simulink model "basic_electricalcircuit"  (R2019a)
settings: Solver=VariableStepAuto  StartTime=0.0  StopTime=0.01  RelTol=1e-3
libraries: powerlib x5
settings Model: Creator=Deepak  LastModifiedBy=Deepak

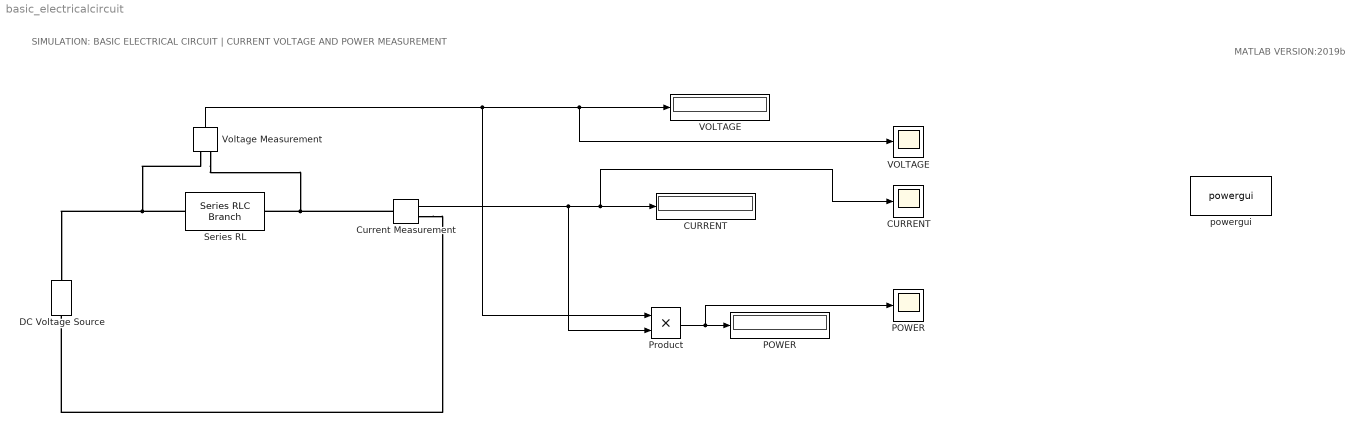
== system basic_electricalcircuit ==
  note: MATLAB VERSION:2019b
  note: SIMULATION: BASIC ELECTRICAL CIRCUIT | CURRENT VOLTAGE AND POWER MEASUREMENT
  CURRENT : Scope
  "CURRENT " : Display
  Current Measurement : powerlib/Measurements/Current Measurement  PhasorSimulation=off  OutputType=Complex  PSBequivalent=0
      settings: SourceProductName=Simscape Electrical
  "DC Voltage Source " : powerlib/Electrical Sources/DC Voltage Source  Amplitude=100  Measurements=None
      settings: SourceProductName=Simscape Electrical
  POWER : Scope
  "POWER " : Display
  Product : Product
  "Series RL " : powerlib/Elements/Series RLC Branch  LConnTagsString=__new0  RConnTagsString=__new0  BranchType=RL  Resistance=10  Inductance=10e-3  SetiL0=off  InitialCurrent=0  Capacitance=1e-6  Setx0=off  InitialVoltage=0  Measurements=None
      settings: SourceProductName=Simscape Electrical
  VOLTAGE : Scope
  "VOLTAGE " : Display
  Voltage Measurement : powerlib/Measurements/Voltage Measurement  PhasorSimulation=off  OutputType=Complex  PSBequivalent=0
      settings: SourceProductName=Simscape Electrical
  powergui : powerlib/powergui  Priority=1  SimulationMode=Continuous  SampleTime=50e-6  frequency=60  Iterations=50  frequencyindice=0  Pbase=100e6  ErrMax=1e-4  UnitsV=kV  UnitsW=MW  buscounter=0  FunctionMessages=off  echomessages=off  EnableUseOfTLC=off  CurrentSourceSwitches=off  DisableSnubberDevices=off  DisableRonSwitches=off  DisableVfSwitches=off  DisplayEquations=off  AutomaticDiscreteSolvers=off  SolverType=Tustin/Backward Euler (TBE)  Interpol=off  ExternalGateDelay=off  methode=off  Ts=100  x0status=blocks  SPID=on  SwTol=0  HookPort=off  NonlinearTolerance=0  nMaxIteration=15  ContinueOnMaxIteration=off  RestoreLinks=warning  ResistiveCurrentMeasurement=off  Frange=[0:2:500]  Ylog=off  Xlog=on  ShowGrid=off  save=off  variable=ZData  structure=0  ZoomFFT=off  StartTime=0.0  cycles=1  DisplayStyle=1  fundamental=60  FreqAxis=off  MaxFrequency=1000  frequencyindicesteady=1  RmsSteady=1  display=off
      settings: SourceProductName=Simscape Electrical
  wires:
  Voltage Measurement/1 -> Product/1, VOLTAGE/1, "VOLTAGE "/1
  Current Measurement/1 -> Product/2, CURRENT/1, "CURRENT "/1
  Product/1 -> POWER/1, "POWER "/1
  connections:
  "Series RL "/LConn1 -- Voltage Measurement/LConn1 -- "DC Voltage Source "/RConn1
  Current Measurement/LConn1 -- Voltage Measurement/LConn2 -- "Series RL "/RConn1
  Current Measurement/RConn1 -- "DC Voltage Source "/LConn1
